simulink model "Model_with_cruise_control"  (R2025a)
settings: Solver=VariableStepAuto  StartTime=0.0  StopTime=20  RelTol=1e-3
values from neighbouring files (symbols this model uses):
  g = 9.8    [LQR.m]
  I = (m*l^2)/3    (= 0.0766666666667)    [LQR.m]
  K = lqr(A, B, Q, R)    [LQR.m]
  l = 1    [LQR.m]
  L = 0.5    [LQR.m]    (also in My_equation_simulation.m; equations.m = 1; simulation.m)
  M = 2.4    [LQR.m]
  m = 0.23    [LQR.m]
settings Model: Creator=Kush  LastModifiedBy=Kush

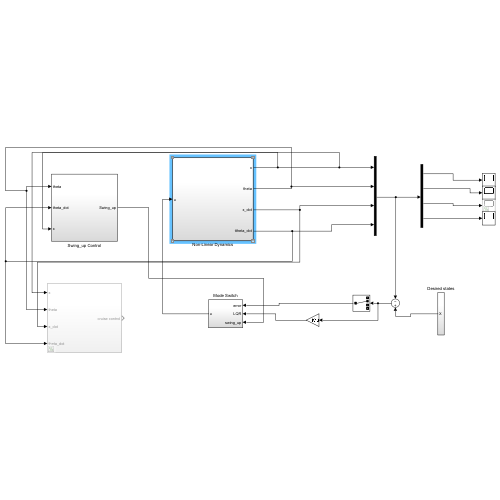
[thumbnail: Simulink's stored preview of the top-level diagram]
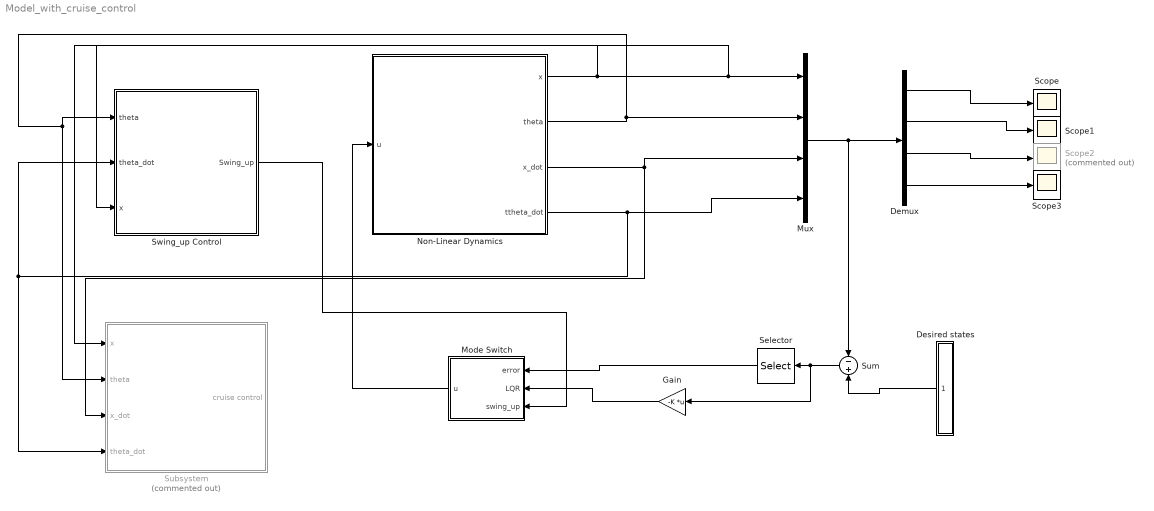
== system Model_with_cruise_control ==
  Demux : Demux
  Desired states : Subsystem
  Gain : Gain  Gain=-K  Multiplication=Matrix(K*u)
  Mode Switch : Subsystem
  Mux : Mux
  Non-Linear Dynamics : Subsystem
  Scope : Scope
      settings: ActiveDisplayYMinimum=-7.9003995931366235  ActiveDisplayYMaximum=2.005222147601597
  Scope1 : Scope
      settings: SampleTime=0.01  ActiveDisplayYMinimum=-3171.3497934475877  ActiveDisplayYMaximum=3076.816580126309
  Scope2 : Scope  Commented=on
      settings: ActiveDisplayYMinimum=-1  ActiveDisplayYMaximum=1  DataLoggingVariableName=ScopeData2
  Scope3 : Scope
      settings: ActiveDisplayYMinimum=-1  ActiveDisplayYMaximum=1  DataLoggingVariableName=ScopeData3
  Selector : Selector  InputPortWidth=4  IndexOptions=Index vector (dialog)  Indices=2  OutputSizes=1
  Subsystem : Subsystem  Commented=on
  Sum : Sum  Inputs=-|+
  Swing_up Control : Subsystem
  wires:
  Non-Linear Dynamics/1(x) -> Swing_up Control/3(x), Subsystem/1(x), Mux/1
  Non-Linear Dynamics/3(x_dot) -> Subsystem/3(x_dot), Mux/3
  Non-Linear Dynamics/4(ttheta_dot) -> Swing_up Control/2(theta_dot), Subsystem/4(theta_dot), Mux/4
  Mux/1 -> Demux/1, Sum/1
  Desired states/1(X) -> Sum/2
  Sum/1 -> Gain/1, Selector/1
  Selector/1 -> Mode Switch/1(error)
  Gain/1 -> Mode Switch/2(LQR)
  Demux/1 -> Scope/1
  Demux/3 -> Scope2/1
  Demux/4 -> Scope3/1
  Swing_up Control/1(Swing_up) -> Mode Switch/3(swing_up)
  Mode Switch/1(u) -> Non-Linear Dynamics/1(u)
  Demux/2 -> Scope1/1
  Non-Linear Dynamics/2(theta) -> Mux/2, Subsystem/2(theta), Swing_up Control/1(theta)

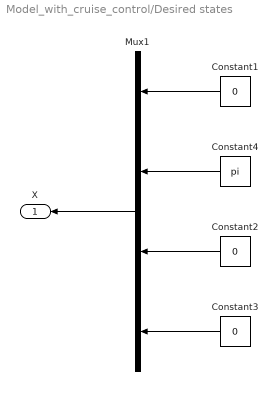
== system Model_with_cruise_control/Desired states ==
  Constant1 : Constant  Value=0
  Constant2 : Constant  Value=0
  Constant3 : Constant  Value=0
  Constant4 : Constant  Value=pi
  Mux1 : Mux
  X : Outport
  wires:
  Constant2/1 -> Mux1/3
  Constant1/1 -> Mux1/1
  Constant3/1 -> Mux1/4
  Constant4/1 -> Mux1/2
  Mux1/1 -> X/1

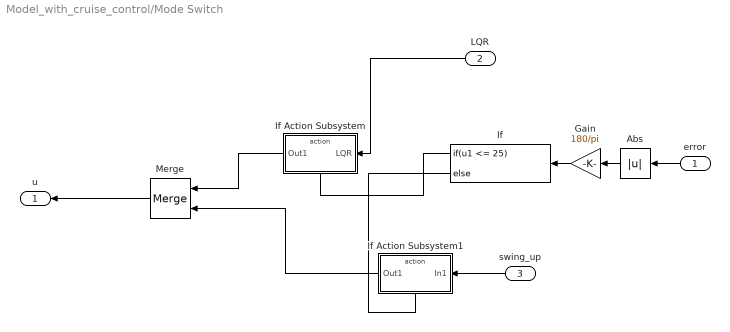
== system Model_with_cruise_control/Mode Switch ==
  error : Inport
  LQR : Inport  Port=2
  swing_up : Inport  Port=3
  Abs : Abs  SaturateOnIntegerOverflow=off
  Gain : Gain  Gain=180/pi
  If : If  IfExpression=u1 <= 25
  If Action Subsystem : Subsystem  TreatAsAtomicUnit=on
  If Action Subsystem1 : Subsystem  TreatAsAtomicUnit=on
  Merge : Merge
  u : Outport
  wires:
  If Action Subsystem1/1(Out1) -> Merge/2
  Gain/1 -> If/1
  If/1 -> If Action Subsystem/Action
  swing_up/1 -> If Action Subsystem1/1(In1)
  error/1 -> Abs/1
  Abs/1 -> Gain/1
  If Action Subsystem/1(Out1) -> Merge/1
  Merge/1 -> u/1
  If/2 -> If Action Subsystem1/Action
  LQR/1 -> If Action Subsystem/1(LQR)

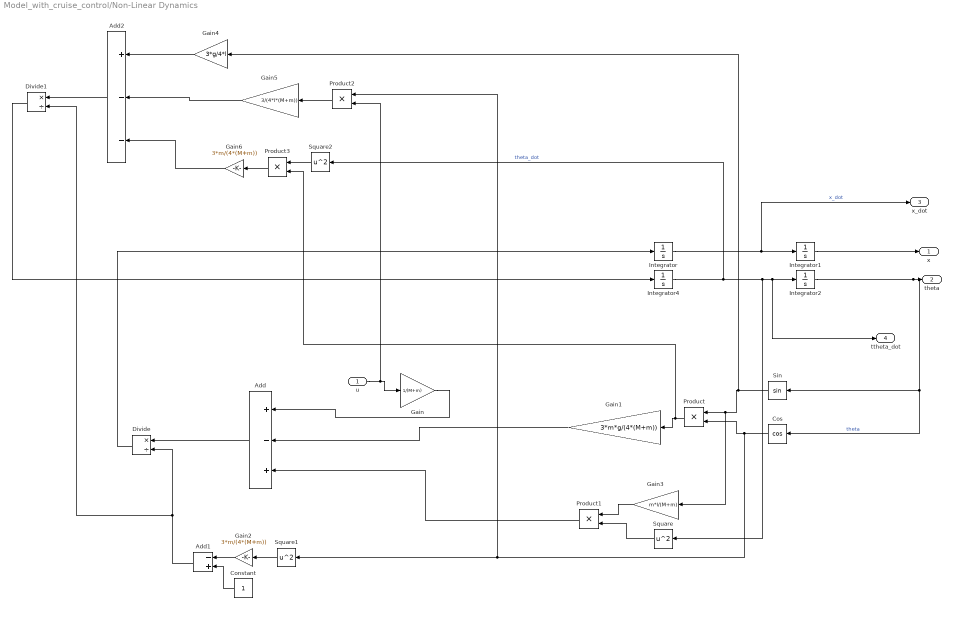
== system Model_with_cruise_control/Non-Linear Dynamics ==
  u : Inport
  Add : Sum  Inputs=+-+
  Add1 : Sum  Inputs=-+
  Add2 : Sum  Inputs=+--
  Constant : Constant
  Cos : Trigonometry  Operator=cos
  Divide : Product  Inputs=*/
  Divide1 : Product  Inputs=*/
  Gain : Gain  Gain=1/(M+m)
  Gain1 : Gain  Gain=3*m*g/(4*(M+m))
  Gain2 : Gain  Gain=3*m/(4*(M+m))
  Gain3 : Gain  Gain=m*l/(M+m)
  Gain4 : Gain  Gain=3*g/4*l
  Gain5 : Gain  Gain=3/(4*l*(M+m))
  Gain6 : Gain  Gain=3*m/(4*(M+m))
  Integrator : Integrator
  Integrator1 : Integrator
  Integrator2 : Integrator  InitialCondition=1*(pi/180)
  Integrator4 : Integrator
  Product{,1..3} (4 alike) : Product
  Sin : Trigonometry
  Square : Math  Operator=square
  Square1 : Math  Operator=square
  Square2 : Math  Operator=square
  x : Outport
  theta : Outport  Port=2
  x_dot : Outport  Port=3
  ttheta_dot : Outport  Port=4
  wires:
  Constant/1 -> Add1/2
  Product2/1 -> Gain5/1
  Gain6/1 -> Add2/3
  Gain5/1 -> Add2/2
  Add1/1 -> Divide1/2, Divide/2
  Gain3/1 -> Product1/1
  Add2/1 -> Divide1/1
  Square2/1 -> Product3/1
  Gain4/1 -> Add2/1
  Product/1 -> Product3/2, Gain1/1
  Product1/1 -> Add/3
  Cos/1 -> Product2/1, Square1/1, Product/2
  Divide1/1 -> Integrator4/1
  u/1 -> Product2/2, Gain/1
  Product3/1 -> Gain6/1
  Square1/1 -> Gain2/1
  Gain1/1 -> Add/2
  Square/1 -> Product1/2
  Gain/1 -> Add/1
  Add/1 -> Divide/1
  Sin/1 -> Gain4/1, Gain3/1, Product/1
  Gain2/1 -> Add1/1
  Integrator4/1 -> Square2/1, Square/1, ttheta_dot/1, Integrator2/1  "theta_dot"
  Divide/1 -> Integrator/1
  Integrator2/1 -> Cos/1, Sin/1, theta/1  "theta"
  Integrator/1 -> x_dot/1, Integrator1/1  "x_dot"
  Integrator1/1 -> x/1

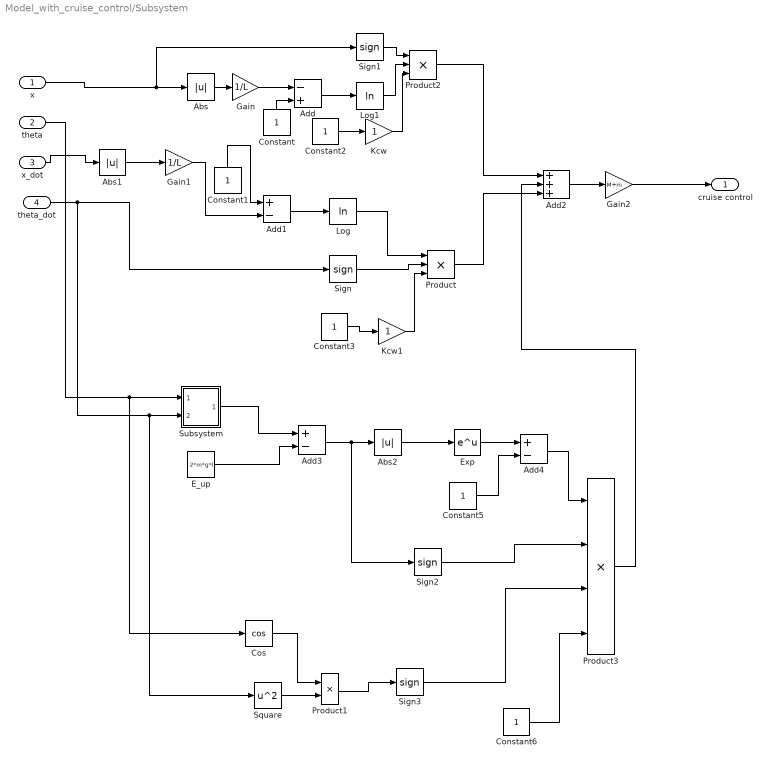
== system Model_with_cruise_control/Subsystem ==
  x : Inport
  theta : Inport  Port=2
  x_dot : Inport  Port=3
  theta_dot : Inport  Port=4
  Abs : Abs  SaturateOnIntegerOverflow=off
  Abs1 : Abs  SaturateOnIntegerOverflow=off
  Abs2 : Abs  SaturateOnIntegerOverflow=off
  Add : Sum  Inputs=-+
  Add1 : Sum  Inputs=+-
  Add2 : Sum  Inputs=+++
  Add3 : Sum  Inputs=+-
  Add4 : Sum  Inputs=+-
  Constant{,1..3,5..6} (6 alike) : Constant
  Cos : Trigonometry  Operator=cos
  E_up : Constant  Value=2*m*g*l
  Exp : Math
  Gain : Gain  Gain=1/L
  Gain1 : Gain  Gain=1/L
  Gain2 : Gain  Gain=M+m
  Kcw : Gain
  Kcw1 : Gain
  Log : Math  Operator=log
  Log1 : Math  Operator=log
  Product : Product  Inputs=3
  Product1 : Product
  Product2 : Product  Inputs=3
  Product3 : Product  Inputs=4
  Sign{,1..3} (4 alike) : Signum
  Square : Math  Operator=square
  Subsystem : Subsystem
  cruise control : Outport
  wires:
  Log1/1 -> Product2/2
  Sign1/1 -> Product2/1
  Constant/1 -> Add/2
  Gain/1 -> Add/1
  Add/1 -> Log1/1
  Abs/1 -> Gain/1
  Kcw/1 -> Product2/3
  x/1 -> Sign1/1, Abs/1
  x_dot/1 -> Abs1/1
  Abs1/1 -> Gain1/1
  Gain1/1 -> Add1/2
  Constant1/1 -> Add1/1
  Add1/1 -> Log/1
  Log/1 -> Product/1
  Sign/1 -> Product/2
  Constant2/1 -> Kcw/1
  Constant3/1 -> Kcw1/1
  Kcw1/1 -> Product/3
  Product2/1 -> Add2/1
  Product/1 -> Add2/3
  theta/1 -> Cos/1, Subsystem/1(In1)
  Subsystem/1(Erp) -> Add3/1
  E_up/1 -> Add3/2
  Add3/1 -> Sign2/1, Abs2/1
  Abs2/1 -> Exp/1
  Exp/1 -> Add4/1
  Constant5/1 -> Add4/2
  theta_dot/1 -> Square/1, Subsystem/2(In2), Sign/1
  Product1/1 -> Sign3/1
  Cos/1 -> Product1/1
  Square/1 -> Product1/2
  Add4/1 -> Product3/1
  Sign2/1 -> Product3/2
  Sign3/1 -> Product3/3
  Constant6/1 -> Product3/4
  Product3/1 -> Add2/2
  Add2/1 -> Gain2/1
  Gain2/1 -> cruise control/1

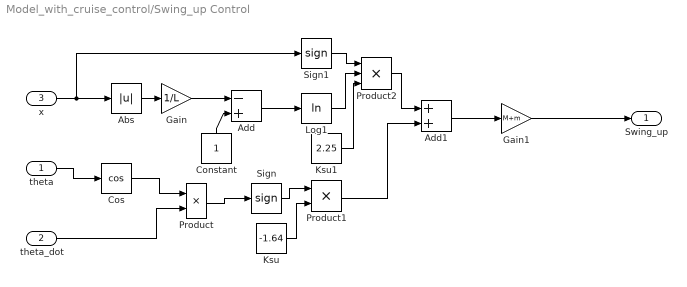
== system Model_with_cruise_control/Swing_up Control ==
  theta : Inport
  theta_dot : Inport  Port=2
  x : Inport  Port=3
  Abs : Abs  SaturateOnIntegerOverflow=off
  Add : Sum  Inputs=-+
  Add1 : Sum
  Constant : Constant
  Cos : Trigonometry  Operator=cos
  Gain : Gain  Gain=1/L
  Gain1 : Gain  Gain=M+m
  Ksu : Constant  Value=-1.64
  Ksu1 : Constant  Value=2.25
  Log1 : Math  Operator=log
  Product : Product
  Product1 : Product
  Product2 : Product  Inputs=3
  Sign : Signum
  Sign1 : Signum
  Swing_up : Outport
  wires:
  Gain1/1 -> Swing_up/1
  theta_dot/1 -> Product/2
  theta/1 -> Cos/1
  Cos/1 -> Product/1
  Product/1 -> Sign/1
  Sign/1 -> Product1/1
  Ksu/1 -> Product1/2
  x/1 -> Sign1/1, Abs/1
  Abs/1 -> Gain/1
  Gain/1 -> Add/1
  Constant/1 -> Add/2
  Add/1 -> Log1/1
  Sign1/1 -> Product2/1
  Log1/1 -> Product2/2
  Ksu1/1 -> Product2/3
  Product2/1 -> Add1/1
  Product1/1 -> Add1/2
  Add1/1 -> Gain1/1

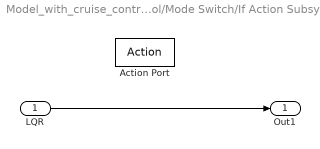
== system Model_with_cruise_control/Mode Switch/If Action Subsystem ==
  LQR : Inport
  Action Port : ActionPort  ActionPortLabel=if(u1 <= 25)
  Out1 : Outport
  wires:
  LQR/1 -> Out1/1

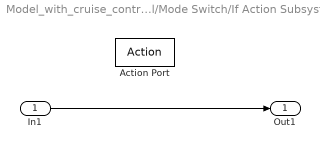
== system Model_with_cruise_control/Mode Switch/If Action Subsystem1 ==
  In1 : Inport
  Action Port : ActionPort  ActionPortLabel=else
  Out1 : Outport
  wires:
  In1/1 -> Out1/1

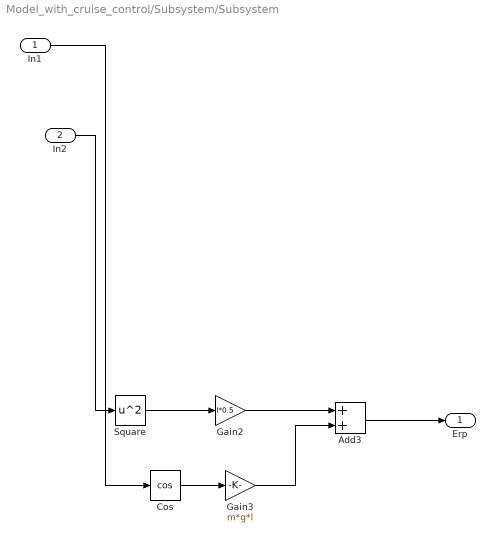
== system Model_with_cruise_control/Subsystem/Subsystem ==
  In1 : Inport
  In2 : Inport  Port=2
  Add3 : Sum
  Cos : Trigonometry  Operator=cos
  Gain2 : Gain  Gain=I*0.5
  Gain3 : Gain  Gain=m*g*l
  Square : Math  Operator=square
  Erp : Outport
  wires:
  Gain2/1 -> Add3/1
  Gain3/1 -> Add3/2
  Add3/1 -> Erp/1
  Square/1 -> Gain2/1
  Cos/1 -> Gain3/1
  In2/1 -> Square/1
  In1/1 -> Cos/1
